simulink model "model_report_gutman_bandwidth_roll"  (R2018b)
settings: Solver=VariableStepAuto  StartTime=0.0  StopTime=10.0  RelTol=1e-3
values from neighbouring files (symbols this model uses):
  A = [0 g/h ; 1 0]    [report_gutman.m]
  B = [1 ; 0]    [report_gutman.m]
  C = [C1*v C2*v^2]    [report_gutman.m]
  C1 = a/(b*h)    (= 0.872633942894)    [report_gutman.m]
  C2 = 1/(b*h)    (= 1.75792494539)    [report_gutman.m]
  D = 0    [report_gutman.m]
  D_steering_position = 0    [report_gutman.m]
  g = 9.81    [report_gutman.m]
  h = figure    [plot_disturbances_bike.m]    (also in report_gutman.m = 0.5195)
  I_steering_position = 30    [report_gutman.m]
  initial_roll = deg2rad(2)    [report_gutman.m]
  initial_rollrate = deg2rad(0)    [report_gutman.m]
  K_feedforward_steering = 0    [report_gutman.m]
  m = 45    [report_gutman.m]
  num_tf_steering = [253.4]    [report_gutman.m]
  P_steering_position = 30    [report_gutman.m]
  Ts = 0.01    [report_gutman.m]
  v = 4    [report_gutman.m]
undefined symbols (not defined in the file or in its folder): ba, bb, lqr_gains, velocity_lqr
libraries: simulink_extras x8, simulink x1
settings Model: Creator=maximef  LastModifiedBy=maximef

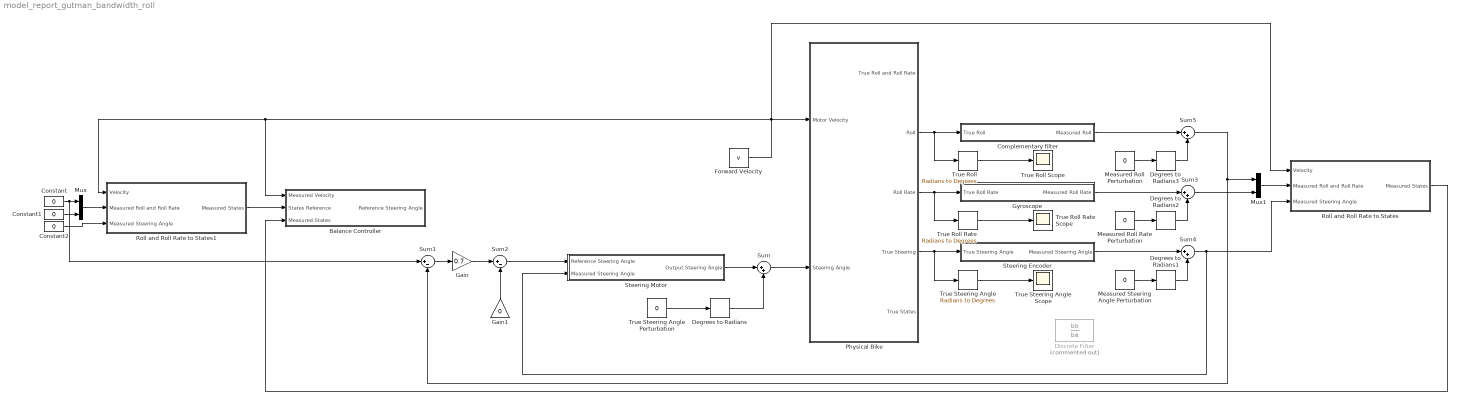
== system model_report_gutman_bandwidth_roll ==
  Balance Controller : Subsystem  SystemSampleTime=Ts
  Complementary filter : Subsystem  TreatAsAtomicUnit=on  SystemSampleTime=Ts
  Constant : Constant  Value=0
  Constant1 : Constant  Value=0
  Constant2 : Constant  Value=0
  Degrees to Radians{,1..3} (4 alike) : simulink_extras/Transformations/Degrees to Radians
  Discrete Filter : DiscreteFilter  Commented=on  Numerator=bb  Denominator=ba
  Forward Velocity : Constant  Value=v
  Gain : Gain  Gain=0.7
  Gain1 : Gain  Gain=0
  Gyroscope : Subsystem  TreatAsAtomicUnit=on  SystemSampleTime=Ts
  Measured Roll Perturbation : Constant  Value=0
  Measured Roll Rate Perturbation : Constant  Value=0
  Measured Steering Angle Perturbation : Constant  Value=0
  Mux : Mux  Inputs=2
  Mux1 : Mux  Inputs=2
  Physical Bike : Subsystem
  Roll and Roll Rate to States : Subsystem
  Roll and Roll Rate to States1 : Subsystem
  Steering Encoder : Subsystem  TreatAsAtomicUnit=on  SystemSampleTime=Ts
  Steering Motor : Subsystem
  Sum{,3..5} (4 alike) : Sum  Inputs=|++
  Sum1 : Sum  Inputs=|+-
  Sum2 : Sum  Inputs=|+-
  True Roll : simulink_extras/Transformations/Radians to Degrees
  True Roll Rate : simulink_extras/Transformations/Radians to Degrees
  True Roll Rate Scope : Scope
  True Roll Scope : Scope
  True Steering Angle : simulink_extras/Transformations/Radians to Degrees
  True Steering Angle Perturbation : Constant  Value=0
  True Steering Angle Scope : Scope
  wires:
  True Roll Rate/1 -> True Roll Rate Scope/1
  Physical Bike/4(True Steering) -> Steering Encoder/1(True Steering Angle), True Steering Angle/1
  Roll and Roll Rate to States1/1(Measured States) -> Balance Controller/2(States Reference)
  Measured Roll Rate Perturbation/1 -> Degrees to Radians2/1
  Physical Bike/3(Roll Rate) -> Gyroscope/1(True Roll Rate), True Roll Rate/1
  Gyroscope/1(Measured Roll Rate) -> Sum3/1
  Sum3/1 -> Mux1/2
  True Steering Angle/1 -> True Steering Angle Scope/1
  Complementary filter/1(Measured Roll) -> Sum5/1
  Measured Steering Angle Perturbation/1 -> Degrees to Radians1/1
  Sum5/1 -> Sum1/2, Mux1/1
  True Steering Angle Perturbation/1 -> Degrees to Radians/1
  Degrees to Radians1/1 -> Sum4/2
  Roll and Roll Rate to States/1(Measured States) -> Balance Controller/3(Measured States)
  Measured Roll Perturbation/1 -> Degrees to Radians3/1
  Degrees to Radians3/1 -> Sum5/2
  Physical Bike/2(Roll) -> Complementary filter/1(True Roll), True Roll/1
  Steering Motor/1(Output Steering Angle) -> Sum/1
  Sum/1 -> Physical Bike/2(Steering Angle)
  Gain/1 -> Sum2/1
  True Roll/1 -> True Roll Scope/1
  Mux1/1 -> Roll and Roll Rate to States/2(Measured Roll and Roll Rate)
  Sum1/1 -> Gain/1
  Degrees to Radians/1 -> Sum/2
  Sum4/1 -> Steering Motor/2(Measured Steering Angle), Roll and Roll Rate to States/3(Measured Steering Angle)
  Constant/1 -> Sum1/1, Mux/1
  Gain1/1 -> Sum2/2
  Forward Velocity/1 -> Roll and Roll Rate to States/1(Velocity), Roll and Roll Rate to States1/1(Velocity), Balance Controller/1(Measured Velocity), Physical Bike/1(Motor Velocity)
  Sum2/1 -> Steering Motor/1(Reference Steering Angle)
  Degrees to Radians2/1 -> Sum3/2
  Steering Encoder/1(Measured Steering Angle) -> Sum4/1
  Mux/1 -> Roll and Roll Rate to States1/2(Measured Roll and Roll Rate)
  Constant1/1 -> Mux/2
  Constant2/1 -> Roll and Roll Rate to States1/3(Measured Steering Angle)

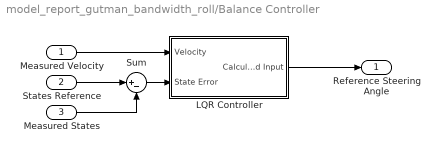
== system model_report_gutman_bandwidth_roll/Balance Controller ==
  Measured Velocity : Inport
  States Reference : Inport  Port=2
  Measured States : Inport  Port=3
  LQR Controller : Subsystem  TreatAsAtomicUnit=on  SystemSampleTime=Ts
  Sum : Sum  Inputs=|+-
  Reference Steering Angle : Outport
  wires:
  Sum/1 -> LQR Controller/2(State Error)
  Measured States/1 -> Sum/2
  LQR Controller/1(Calculated Input) -> Reference Steering Angle/1
  Measured Velocity/1 -> LQR Controller/1(Velocity)
  States Reference/1 -> Sum/1

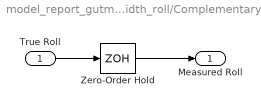
== system model_report_gutman_bandwidth_roll/Complementary filter ==
  True Roll : Inport
  Zero-Order Hold : ZeroOrderHold  SampleTime=Ts
  Measured Roll : Outport
  wires:
  True Roll/1 -> Zero-Order Hold/1
  Zero-Order Hold/1 -> Measured Roll/1

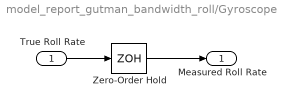
== system model_report_gutman_bandwidth_roll/Gyroscope ==
  True Roll Rate : Inport
  Zero-Order Hold : ZeroOrderHold  SampleTime=Ts
  Measured Roll Rate : Outport
  wires:
  True Roll Rate/1 -> Zero-Order Hold/1
  Zero-Order Hold/1 -> Measured Roll Rate/1

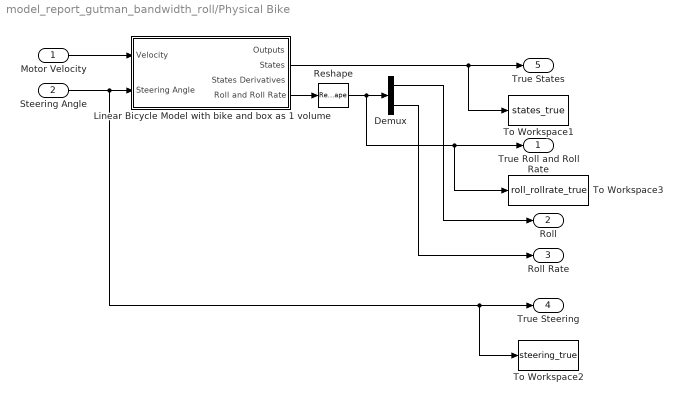
== system model_report_gutman_bandwidth_roll/Physical Bike ==
  Motor Velocity : Inport
  Steering Angle : Inport  Port=2
  Demux : Demux  Outputs=2
  Linear Bicycle Model with bike and box as 1 volume : Subsystem
  Reshape : Reshape
  To Workspace1 : ToWorkspace  VariableName=states_true  SaveFormat=Timeseries  SampleTime=-1
  To Workspace2 : ToWorkspace  VariableName=steering_true  SaveFormat=Timeseries  SampleTime=-1
  To Workspace3 : ToWorkspace  VariableName=roll_rollrate_true  SaveFormat=Timeseries  SampleTime=-1
  True Roll and Roll Rate : Outport
  Roll : Outport  Port=2
  Roll Rate : Outport  Port=3
  True Steering : Outport  Port=4
  True States : Outport  Port=5
  wires:
  Steering Angle/1 -> To Workspace2/1, True Steering/1, Linear Bicycle Model with bike and box as 1 volume/2(Steering Angle)
  Motor Velocity/1 -> Linear Bicycle Model with bike and box as 1 volume/1(Velocity)
  Linear Bicycle Model with bike and box as 1 volume/2(States) -> To Workspace1/1, True States/1
  Demux/1 -> Roll/1
  Linear Bicycle Model with bike and box as 1 volume/4(Roll and Roll Rate) -> Reshape/1
  Reshape/1 -> To Workspace3/1, True Roll and Roll Rate/1, Demux/1
  Demux/2 -> Roll Rate/1

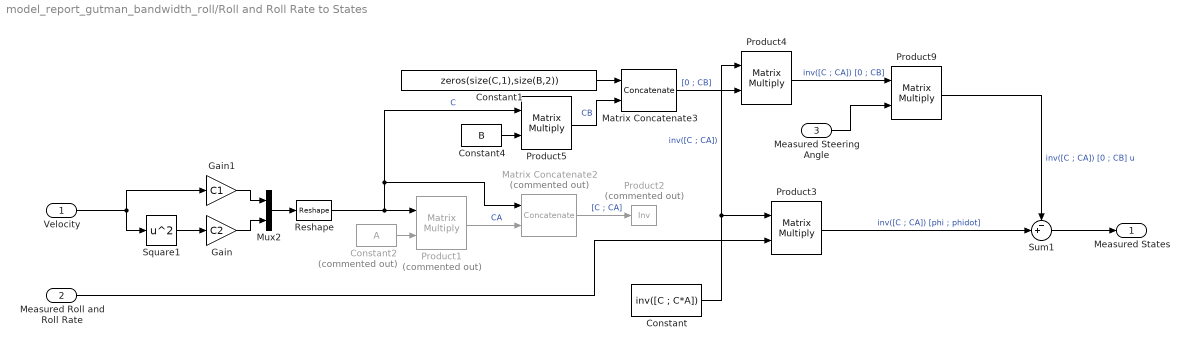
== system model_report_gutman_bandwidth_roll/Roll and Roll Rate to States ==
  Velocity : Inport
  Measured Roll and Roll Rate : Inport  Port=2
  Measured Steering Angle : Inport  Port=3
  Constant : Constant  Value=inv([C ; C*A])
  Constant1 : Constant  Value=zeros(size(C,1),size(B,2))
  Constant2 : Constant  Commented=on  Value=A
  Constant4 : Constant  Value=B
  Gain : Gain  Gain=C2
  Gain1 : Gain  Gain=C1
  Matrix Concatenate2 : Concatenate  Commented=on  Mode=Multidimensional array
  Matrix Concatenate3 : Concatenate  Mode=Multidimensional array
  Mux2 : Mux  Inputs=2
  Product1 : Product  Commented=on  SCDEnableBlockLinearizationSpecification=on  Multiplication=Matrix(*)
  Product2 : Product  Commented=on  SCDEnableBlockLinearizationSpecification=on  Inputs=/  Multiplication=Matrix(*)
  Product{3..5,9} (4 alike) : Product  SCDEnableBlockLinearizationSpecification=on  Multiplication=Matrix(*)
  Reshape : Reshape  OutputDimensionality=Row vector (2-D)
  Square1 : Math  Operator=square  SaturateOnIntegerOverflow=on
  Sum1 : Sum  Inputs=-+|
  Measured States : Outport
  wires:
  Reshape/1 -> Product5/1, Matrix Concatenate2/1, Product1/1  "C"
  Velocity/1 -> Square1/1, Gain1/1
  Square1/1 -> Gain/1
  Gain/1 -> Mux2/2
  Gain1/1 -> Mux2/1
  Mux2/1 -> Reshape/1
  Constant2/1 -> Product1/2
  Matrix Concatenate2/1 -> Product2/1  "[C ; CA]"
  Product1/1 -> Matrix Concatenate2/2  "CA"
  Constant/1 -> Product4/1, Product3/1  "inv([C ; CA])"
  Product3/1 -> Sum1/2  "inv([C ; CA]) [phi ; phidot]"
  Matrix Concatenate3/1 -> Product4/2  "[0 ; CB]"
  Product5/1 -> Matrix Concatenate3/2  "CB"
  Constant4/1 -> Product5/2
  Constant1/1 -> Matrix Concatenate3/1
  Product4/1 -> Product9/1  "inv([C ; CA]) [0 ; CB]"
  Measured Steering Angle/1 -> Product9/2
  Product9/1 -> Sum1/1  "inv([C ; CA]) [0 ; CB] u"
  Sum1/1 -> Measured States/1
  Measured Roll and Roll Rate/1 -> Product3/2

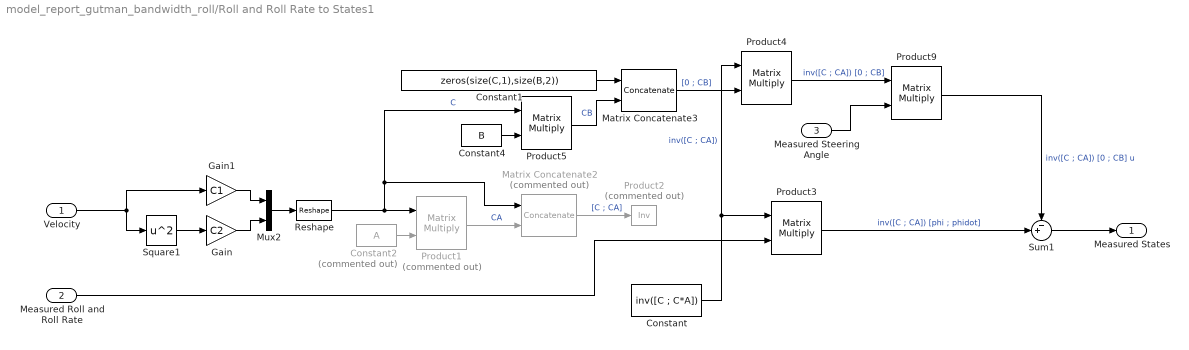
== system model_report_gutman_bandwidth_roll/Roll and Roll Rate to States1 ==
  Velocity : Inport
  Measured Roll and Roll Rate : Inport  Port=2
  Measured Steering Angle : Inport  Port=3
  Constant : Constant  Value=inv([C ; C*A])
  Constant1 : Constant  Value=zeros(size(C,1),size(B,2))
  Constant2 : Constant  Commented=on  Value=A
  Constant4 : Constant  Value=B
  Gain : Gain  Gain=C2
  Gain1 : Gain  Gain=C1
  Matrix Concatenate2 : Concatenate  Commented=on  Mode=Multidimensional array
  Matrix Concatenate3 : Concatenate  Mode=Multidimensional array
  Mux2 : Mux  Inputs=2
  Product1 : Product  Commented=on  SCDEnableBlockLinearizationSpecification=on  Multiplication=Matrix(*)
  Product2 : Product  Commented=on  SCDEnableBlockLinearizationSpecification=on  Inputs=/  Multiplication=Matrix(*)
  Product{3..5,9} (4 alike) : Product  SCDEnableBlockLinearizationSpecification=on  Multiplication=Matrix(*)
  Reshape : Reshape  OutputDimensionality=Row vector (2-D)
  Square1 : Math  Operator=square  SaturateOnIntegerOverflow=on
  Sum1 : Sum  Inputs=-+|
  Measured States : Outport
  wires:
  Reshape/1 -> Product5/1, Matrix Concatenate2/1, Product1/1  "C"
  Velocity/1 -> Square1/1, Gain1/1
  Square1/1 -> Gain/1
  Gain/1 -> Mux2/2
  Gain1/1 -> Mux2/1
  Mux2/1 -> Reshape/1
  Constant2/1 -> Product1/2
  Matrix Concatenate2/1 -> Product2/1  "[C ; CA]"
  Product1/1 -> Matrix Concatenate2/2  "CA"
  Constant/1 -> Product4/1, Product3/1  "inv([C ; CA])"
  Product3/1 -> Sum1/2  "inv([C ; CA]) [phi ; phidot]"
  Matrix Concatenate3/1 -> Product4/2  "[0 ; CB]"
  Product5/1 -> Matrix Concatenate3/2  "CB"
  Constant4/1 -> Product5/2
  Constant1/1 -> Matrix Concatenate3/1
  Product4/1 -> Product9/1  "inv([C ; CA]) [0 ; CB]"
  Measured Steering Angle/1 -> Product9/2
  Product9/1 -> Sum1/1  "inv([C ; CA]) [0 ; CB] u"
  Sum1/1 -> Measured States/1
  Measured Roll and Roll Rate/1 -> Product3/2

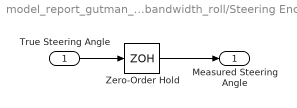
== system model_report_gutman_bandwidth_roll/Steering Encoder ==
  True Steering Angle : Inport
  Zero-Order Hold : ZeroOrderHold  SampleTime=Ts
  Measured Steering Angle : Outport
  wires:
  True Steering Angle/1 -> Zero-Order Hold/1
  Zero-Order Hold/1 -> Measured Steering Angle/1

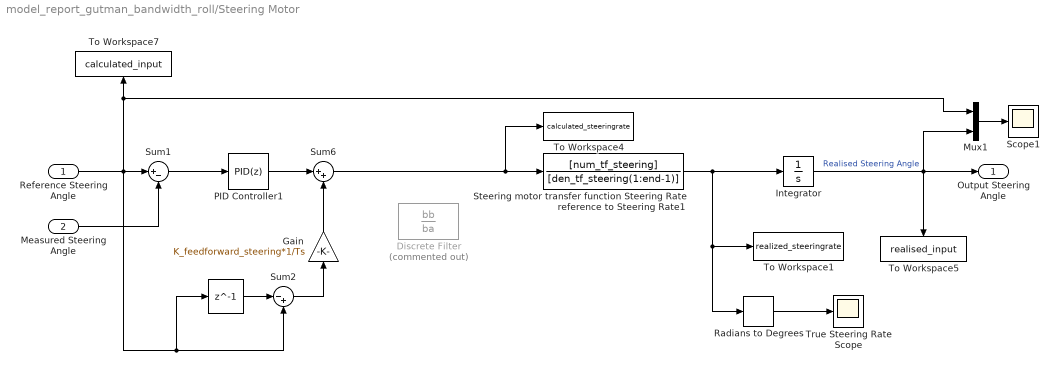
== system model_report_gutman_bandwidth_roll/Steering Motor ==
  Reference Steering Angle : Inport
  Measured Steering Angle : Inport  Port=2
  " " : Delay  DelayLength=1  SampleTime=Ts
  Discrete Filter : DiscreteFilter  Commented=on  Numerator=bb  Denominator=ba
  Gain : Gain  Gain=K_feedforward_steering*1/Ts
  Integrator : Integrator
  Mux1 : Mux  Inputs=2
  PID Controller1 : simulink/Continuous/PID Controller  Controller=PID  Form=Parallel  TimeDomain=Discrete-time  SampleTime=Ts  IntegratorMethod=Forward Euler  FilterMethod=Forward Euler  ControllerParametersSource=internal  P=P_steering_position  I=I_steering_position  D=D_steering_position  UseFilter=off  N=1  TunerSelectOption=Transfer Function Based (PID Tuner App)  InitialConditionSource=internal  InitialConditionForIntegrator=0  InitialConditionForFilter=0  DifferentiatorICPrevScaledInput=0  ExternalReset=none  TrackingMode=off  Kt=1  LimitOutput=off  UpperSaturationLimit=inf  LowerSaturationLimit=-inf  LinearizeAsGain=on  AntiWindupMode=none  Kb=1  POutMin=[]  POutMax=[]  IOutMin=[]  IOutMax=[]  DOutMin=[]  DOutMax=[]  NOutMin=[]  NOutMax=[]  SumOutMin=[]  SumOutMax=[]  SaturationOutMin=[]  SaturationOutMax=[]  PParamMin=[]  PParamMax=[]  IParamMin=[]  IParamMax=[]  DParamMin=[]  DParamMax=[]  NParamMin=[]  NParamMax=[]  KbParamMin=[]  KbParamMax=[]  KtParamMin=[]  KtParamMax=[]  KbOutMin=[]  KbOutMax=[]  KtOutMin=[]  KtOutMax=[]  IntegratorOutMin=[]  IntegratorOutMax=[]  FilterOutMin=[]  FilterOutMax=[]  SumI1OutMin=[]  SumI1OutMax=[]  SumI2OutMin=[]  SumI2OutMax=[]  SumI3OutMin=[]  SumI3OutMax=[]  SumI4OutMin=[]  SumI4OutMax=[]  SumDOutMin=[]  SumDOutMax=[]  DifferentiatorOutMin=[]  DifferentiatorOutMax=[]  FilterDiffOutCoefMin=[]  FilterDiffOutCoefMax=[]  ReciprocalOutMin=[]  ReciprocalOutMax=[]  SumDenOutMin=[]  SumDenOutMax=[]  SumNumOutMin=[]  SumNumOutMax=[]  DivideOutMin=[]  DivideOutMax=[]  IntegratorContinuousStateAttributes=''  IntegratorStateMustResolveToSignalObject=off  IntegratorRTWStateStorageClass=Auto  FilterContinuousStateAttributes=''  FilterStateMustResolveToSignalObject=off  FilterRTWStateStorageClass=Auto  ParallelPVariant=InternalParameters  IdealPVariant=Disabled  IVariant=InternalParameters  DVariant=InternalParameters  IntegratorVariant=Discrete  SatVariant=Disabled  AWVariant=Passthrough  PCopyVariant=Disabled  TRVariant=Disabled  FdbkBlocksVariant=Forward  IdealPFdbkVariant=Disabled  SatFdbkVariant=Disabled  DerivativeFilterVariant=Differentiator  NVariant=Passthrough  NCopyVariant=Disabled_SignalSpec  FilterICVariant=InternalICsDifferentiator  IntegratorICVariant=InternalICs  ExternalResetVariant=Disabled  TRSumVariant=Passthrough  SumFdbkVariant=Disabled  SumVariant=Sum_PID
  Radians to Degrees : simulink_extras/Transformations/Radians to Degrees
  Scope1 : Scope
  Steering motor transfer function Steering Rate reference to Steering Rate1 : TransferFcn  Numerator=[num_tf_steering]  Denominator=[den_tf_steering(1:end-1)]
  Sum1 : Sum  Inputs=|+-
  Sum2 : Sum  Inputs=|-+
  Sum6 : Sum  Inputs=|++
  To Workspace1 : ToWorkspace  VariableName=realized_steeringrate  SaveFormat=Timeseries  SampleTime=-1
  To Workspace4 : ToWorkspace  VariableName=calculated_steeringrate  SaveFormat=Timeseries  SampleTime=-1
  To Workspace5 : ToWorkspace  VariableName=realised_input  SaveFormat=Timeseries  SampleTime=-1
  To Workspace7 : ToWorkspace  VariableName=calculated_input  SaveFormat=Timeseries  SampleTime=Ts
  True Steering Rate Scope : Scope
  Output Steering Angle : Outport
  wires:
  Mux1/1 -> Scope1/1
  Reference Steering Angle/1 -> Mux1/1, To Workspace7/1, Sum1/1, Sum2/2, " "/1
  Measured Steering Angle/1 -> Sum1/2
  " "/1 -> Sum2/1
  Sum2/1 -> Gain/1
  Sum1/1 -> PID Controller1/1
  Integrator/1 -> Output Steering Angle/1, Mux1/2, To Workspace5/1  "Realised Steering Angle"
  PID Controller1/1 -> Sum6/1
  Gain/1 -> Sum6/2
  Steering motor transfer function Steering Rate reference to Steering Rate1/1 -> Integrator/1, Radians to Degrees/1, To Workspace1/1
  Sum6/1 -> Steering motor transfer function Steering Rate reference to Steering Rate1/1, To Workspace4/1
  Radians to Degrees/1 -> True Steering Rate Scope/1

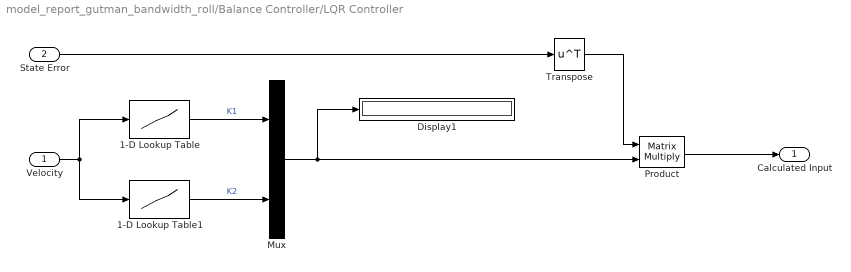
== system model_report_gutman_bandwidth_roll/Balance Controller/LQR Controller ==
  Velocity : Inport
  State Error : Inport  Port=2
  1-D Lookup Table : Lookup_n-D  NumberOfTableDimensions=1  BreakpointsForDimension1=velocity_lqr  BreakpointsForDimension2=velocity_lqr  BreakpointsForDimension3=velocity_lqr  BreakpointsForDimension4=velocity_lqr  Table=lqr_gains(:,2)  InternalRulePriority=Speed  RndMeth=Simplest  InputSameDT=on
  1-D Lookup Table1 : Lookup_n-D  NumberOfTableDimensions=1  BreakpointsForDimension1=velocity_lqr  BreakpointsForDimension2=velocity_lqr  BreakpointsForDimension3=velocity_lqr  BreakpointsForDimension4=velocity_lqr  Table=lqr_gains(:,3)  InternalRulePriority=Speed  RndMeth=Simplest  InputSameDT=on
  Display1 : Display
  Mux : Mux  Inputs=2
  Product : Product  Multiplication=Matrix(*)
  Transpose : Math  Operator=transpose  SaturateOnIntegerOverflow=on
  Calculated Input : Outport
  wires:
  1-D Lookup Table/1 -> Mux/1  "K1"
  1-D Lookup Table1/1 -> Mux/2  "K2"
  Velocity/1 -> 1-D Lookup Table1/1, 1-D Lookup Table/1
  Mux/1 -> Product/2, Display1/1
  Transpose/1 -> Product/1
  Product/1 -> Calculated Input/1
  State Error/1 -> Transpose/1

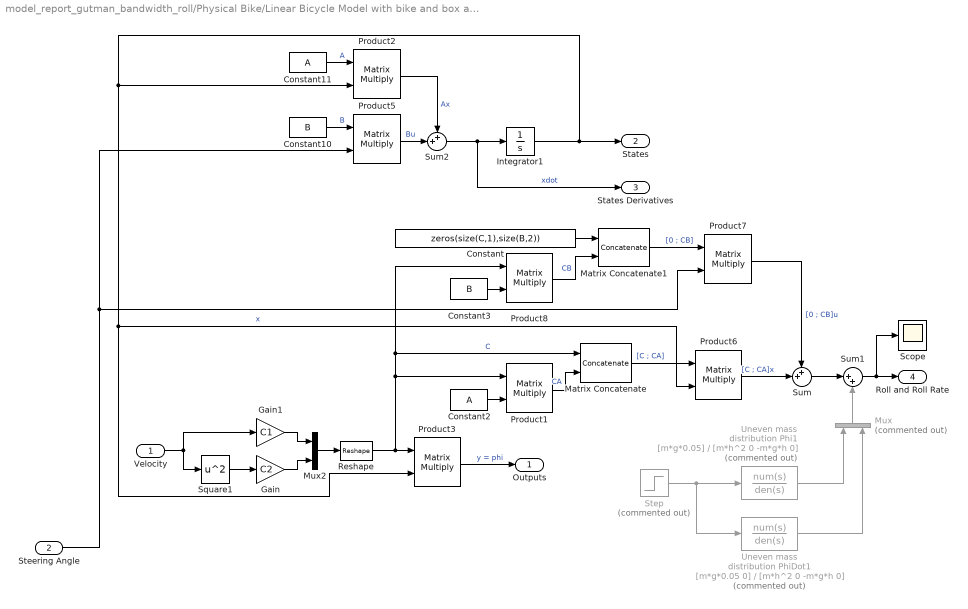
== system model_report_gutman_bandwidth_roll/Physical Bike/Linear Bicycle Model with bike and box as 1 volume ==
  Velocity : Inport
  Steering Angle : Inport  Port=2
  Constant : Constant  Value=zeros(size(C,1),size(B,2))
  Constant10 : Constant  Value=B
  Constant11 : Constant  Value=A
  Constant2 : Constant  Value=A
  Constant3 : Constant  Value=B
  Gain : Gain  Gain=C2
  Gain1 : Gain  Gain=C1
  Integrator1 : Integrator  InitialCondition=[C ; C*A]\[initial_roll ; initial_rollrate]
  Matrix Concatenate : Concatenate  Mode=Multidimensional array
  Matrix Concatenate1 : Concatenate  Mode=Multidimensional array
  Mux : Mux  Commented=on  Inputs=2
  Mux2 : Mux  Inputs=2
  Product{1..3,5..8} (7 alike) : Product  SCDEnableBlockLinearizationSpecification=on  Multiplication=Matrix(*)
  Reshape : Reshape  OutputDimensionality=Row vector (2-D)
  Scope : Scope
  Square1 : Math  Operator=square  SaturateOnIntegerOverflow=on
  Step : Step  Commented=on  Time=0  SampleTime=0
  Sum : Sum  Inputs=++|
  Sum1 : Sum  Inputs=|++
  Sum2 : Sum  Inputs=++|
  Uneven mass distribution Phi1 : TransferFcn  Commented=on  Numerator=[m*g*0.05]  Denominator=[m*h^2 0 -m*g*h 0]
  Uneven mass distribution PhiDot1 : TransferFcn  Commented=on  Numerator=[m*g*0.05 0]  Denominator=[m*h^2 0 -m*g*h 0]
  Outputs : Outport
  States : Outport  Port=2
  States Derivatives : Outport  Port=3
  Roll and Roll Rate : Outport  Port=4
  wires:
  Integrator1/1 -> Product2/2, Product6/2, Product3/2, States/1  "x"
  Product3/1 -> Outputs/1  "y = phi"
  Steering Angle/1 -> Product5/2, Product7/2
  Product2/1 -> Sum2/1  "Ax"
  Mux2/1 -> Reshape/1
  Product5/1 -> Sum2/2  "Bu"
  Sum2/1 -> Integrator1/1, States Derivatives/1  "xdot"
  Constant11/1 -> Product2/1  "A"
  Constant10/1 -> Product5/1  "B"
  Velocity/1 -> Gain1/1, Square1/1
  Square1/1 -> Gain/1
  Reshape/1 -> Product3/1, Product8/1, Matrix Concatenate/1, Product1/1  "C"
  Gain/1 -> Mux2/2
  Gain1/1 -> Mux2/1
  Sum/1 -> Sum1/1
  Constant2/1 -> Product1/2
  Product1/1 -> Matrix Concatenate/2  "CA"
  Matrix Concatenate/1 -> Product6/1  "[C ; CA]"
  Product6/1 -> Sum/2  "[C ; CA]x"
  Product7/1 -> Sum/1  "[0 ; CB]u"
  Matrix Concatenate1/1 -> Product7/1  "[0 ; CB]"
  Product8/1 -> Matrix Concatenate1/2  "CB"
  Constant3/1 -> Product8/2
  Constant/1 -> Matrix Concatenate1/1
  Step/1 -> Uneven mass distribution Phi1/1, Uneven mass distribution PhiDot1/1
  Uneven mass distribution Phi1/1 -> Mux/1
  Sum1/1 -> Scope/1, Roll and Roll Rate/1
  Mux/1 -> Sum1/2
  Uneven mass distribution PhiDot1/1 -> Mux/2
